simulink model "model_dwu"  (R2014b)
settings: Solver=ode45  StartTime=0.0  StopTime=10.0  RelTol=1e-3
values from neighbouring files (symbols this model uses):
  dwu_off = dwu_off_tab(3)    [zad1.m]
  dwu_on = dwu_on_tab(3)    [zad1.m]
  k0 = 2    [zad1.m]
  T1 = 3    [zad1.m]
  T2 = 4    [zad1.m]
  zadana = 5    [zad1.m]
settings Model: Creator=Dyzio  LastModifiedBy=Dyzio

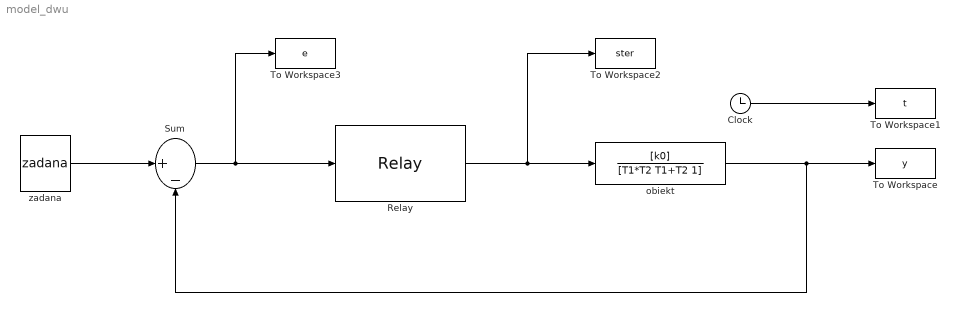
== system model_dwu ==
  Clock : Clock
  Relay : Relay  OnSwitchValue=dwu_on  OffSwitchValue=dwu_off  OnOutputValue=zadana
  Sum : Sum  Inputs=|+-
  To Workspace : ToWorkspace  VariableName=y  SampleTime=-1
  To Workspace1 : ToWorkspace  VariableName=t  SampleTime=-1
  To Workspace2 : ToWorkspace  VariableName=ster  SampleTime=-1
  To Workspace3 : ToWorkspace  VariableName=e  SampleTime=-1
  obiekt : TransferFcn  Numerator=[k0]  Denominator=[T1*T2 T1+T2 1]
  zadana : Constant  Value=zadana
  wires:
  zadana/1 -> Sum/1
  obiekt/1 -> Sum/2, To Workspace/1
  Clock/1 -> To Workspace1/1
  Sum/1 -> To Workspace3/1, Relay/1
  Relay/1 -> To Workspace2/1, obiekt/1
